simulink model "fcn_prb"  (R2020a)
settings: Solver=FixedStepAuto  StartTime=0.0  StopTime=10  FixedStep=0.01  RelTol=1e-3
libraries: androidcommunicationlib x4, androiduilib x1
settings Model: Creator=corte  LastModifiedBy=corte
settings OptimizationCC: EnhancedBackFolding=on  PassReuseOutputArgsAs=Individual arguments  ZeroExternalMemoryAtStartup=off  ZeroInternalMemoryAtStartup=off  MaxStackSize=64  OptimizeBlockOrder=speed  DifferentSizesBufferReuse=on  OptimizationCustomize=off  EfficientTunableParamExpr=on
settings DebuggingCC: ParameterTunabilityLossMsg=error
settings HardwareCC: ProdBitPerPointer=32  ProdBitPerSizeT=32  ProdBitPerPtrDiffT=32  ProdLargestAtomicInteger=Long  ProdLargestAtomicFloat=Double  ProdWordSize=32  ProdHWDeviceType=ARM Compatible->ARM Cortex
settings SFSimCC: MATLABDynamicMemAlloc=off
settings RTWCC: SystemTargetFile=ert.tlc  HardwareBoard=Android Device  TemplateMakefile=ert_default_tmf  RTWVerbose=off  Toolchain=Android SDK/NDK Tools
settings CodeAppCC: ForceParamTrailComments=on  IgnoreCustomStorageClasses=off  OperatorAnnotations=on  SimulinkDataObjDesc=on  SFDataObjDesc=on  InsertBlockDesc=on
settings ERTTargetCC: SupportContinuousTime=on

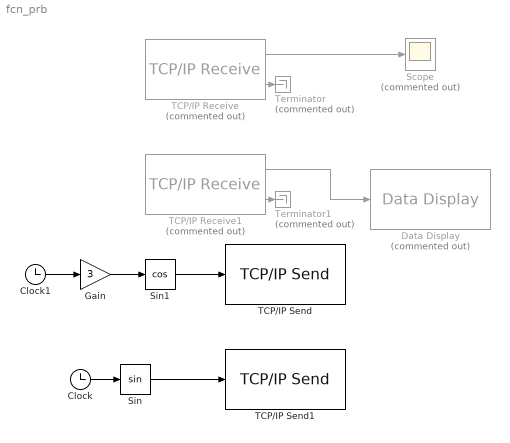
== system fcn_prb ==
  Clock : Clock
  Clock1 : Clock
  Data Display : androiduilib/Data Display  Commented=on  DataDisplayId=fcn_prb/Data_Display  Format=Float  Precision=6  SimulateUsing=Code generation  blockPlatform=Android
      settings: SourceProductBaseCode=ANDROID
  Gain : Gain  Gain=3
  Scope : Scope  Commented=on
  Sin : Trigonometry
  Sin1 : Trigonometry  Operator=cos
  TCP/IP Receive : androidcommunicationlib/TCP//IP Receive  Commented=on  TCPReceiveId=fcn_prb/TCP//IP_Receive  Mode_=Client  LocalServerPort_=25000  RemoteAddr_=192.168.0.15  RemoteServerPort_=25000  DataType_=double  DataSize_=1  SampleTime_=0.01  SimulateUsing=Code generation  ClientPortBindingSelection_=off  ClientPortToBind_=35000  BlockingMode_=off  BlockTimeout_=0.1
      settings: SourceProductBaseCode=ANDROID
  TCP/IP Receive1 : androidcommunicationlib/TCP//IP Receive  Commented=on  TCPReceiveId=fcn_prb/TCP//IP_Receive1  Mode_=Client  LocalServerPort_=25000  RemoteAddr_=192.168.0.15  RemoteServerPort_=25001  DataType_=double  DataSize_=1  SampleTime_=0.01  SimulateUsing=Code generation  ClientPortBindingSelection_=off  ClientPortToBind_=35000  BlockingMode_=off  BlockTimeout_=0.1
      settings: SourceProductBaseCode=ANDROID
  TCP/IP Send : androidcommunicationlib/TCP//IP Send  TCPSendId=fcn_prb/TCP//IP_Send  Mode_=Server  LocalServerPort_=25000  RemoteAddr_=192.168.0.15  RemoteServerPort_=25000  SimulateUsing=Code generation  ClientPortBindingSelection_=off  ClientPortToBind_=35000  BlockingMode_=off  BlockTimeout_=0.1
      settings: SourceProductBaseCode=ANDROID
  TCP/IP Send1 : androidcommunicationlib/TCP//IP Send  TCPSendId=fcn_prb/TCP//IP_Send1  Mode_=Server  LocalServerPort_=25001  RemoteAddr_=192.168.0.15  RemoteServerPort_=25000  SimulateUsing=Code generation  ClientPortBindingSelection_=off  ClientPortToBind_=35000  BlockingMode_=off  BlockTimeout_=0.1
      settings: SourceProductBaseCode=ANDROID
  Terminator : Terminator  Commented=on
  Terminator1 : Terminator  Commented=on
  wires:
  TCP/IP Receive/2 -> Terminator/1
  Clock/1 -> Sin/1
  Sin/1 -> TCP/IP Send1/1
  Clock1/1 -> Gain/1
  TCP/IP Receive/1 -> Scope/1
  TCP/IP Receive1/2 -> Terminator1/1
  TCP/IP Receive1/1 -> Data Display/1
  Gain/1 -> Sin1/1
  Sin1/1 -> TCP/IP Send/1
